simulink model "StateSpaceToScopes"  (R2023b)
settings: Solver=VariableStepAuto  StartTime=0.0  StopTime=100  RelTol=1e-3
undefined symbols (not defined in the file or in its folder): A_1, A_2, A_3, A_4, A_5, A_6, A_7, A_8, B_1, B_2, B_3, B_4, B_5, B_6, B_7, B_8, C_1, C_2, C_3, C_4, C_5, C_6, C_7, C_8, D_1, D_2, D_3, D_4, D_5, D_6, D_7, D_8, F1, F2, F3, F4, F5, F6, F7, F8, G1, G2, G3, G4, G5, G6, G7, G8, H1, H2, H3, H4, H5, H6, H7, H8, J1, J2, J3, J4 ... (+4)
settings Model: Creator=Alex  LastModifiedBy=Alex

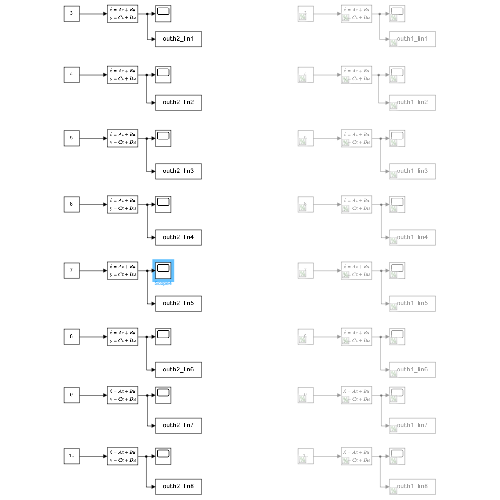
[thumbnail: Simulink's stored preview of the top-level diagram]
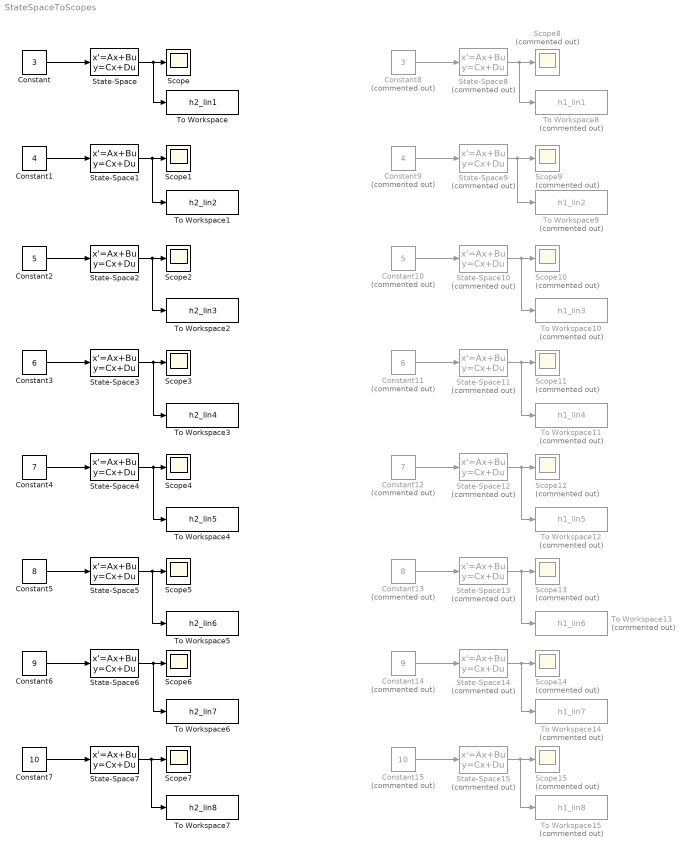
== system StateSpaceToScopes ==
  Constant : Constant  Value=3
  Constant1 : Constant  Value=4
  Constant10 : Constant  Commented=on  Value=5
  Constant11 : Constant  Commented=on  Value=6
  Constant12 : Constant  Commented=on  Value=7
  Constant13 : Constant  Commented=on  Value=8
  Constant14 : Constant  Commented=on  Value=9
  Constant15 : Constant  Commented=on  Value=10
  Constant2 : Constant  Value=5
  Constant3 : Constant  Value=6
  Constant4 : Constant  Value=7
  Constant5 : Constant  Value=8
  Constant6 : Constant  Value=9
  Constant7 : Constant  Value=10
  Constant8 : Constant  Commented=on  Value=3
  Constant9 : Constant  Commented=on  Value=4
  Scope{,1..7} (8 alike) : Scope
  Scope{8..15} (8 alike) : Scope  Commented=on
  State-Space : StateSpace  A=F1  B=G1  C=H1  D=J1  InitialCondition=0
  State-Space1 : StateSpace  A=F2  B=G2  C=H2  D=J2  InitialCondition=0
  State-Space10 : StateSpace  Commented=on  A=A_3  B=B_3  C=C_3  D=D_3  InitialCondition=0
  State-Space11 : StateSpace  Commented=on  A=A_4  B=B_4  C=C_4  D=D_4  InitialCondition=0
  State-Space12 : StateSpace  Commented=on  A=A_5  B=B_5  C=C_5  D=D_5  InitialCondition=0
  State-Space13 : StateSpace  Commented=on  A=A_6  B=B_6  C=C_6  D=D_6  InitialCondition=0
  State-Space14 : StateSpace  Commented=on  A=A_7  B=B_7  C=C_7  D=D_7  InitialCondition=0
  State-Space15 : StateSpace  Commented=on  A=A_8  B=B_8  C=C_8  D=D_8  InitialCondition=0
  State-Space2 : StateSpace  A=F3  B=G3  C=H3  D=J3  InitialCondition=0
  State-Space3 : StateSpace  A=F4  B=G4  C=H4  D=J4  InitialCondition=0
  State-Space4 : StateSpace  A=F5  B=G5  C=H5  D=J5  InitialCondition=0
  State-Space5 : StateSpace  A=F6  B=G6  C=H6  D=J6  InitialCondition=0
  State-Space6 : StateSpace  A=F7  B=G7  C=H7  D=J7  InitialCondition=0
  State-Space7 : StateSpace  A=F8  B=G8  C=H8  D=J8  InitialCondition=0
  State-Space8 : StateSpace  Commented=on  A=A_1  B=B_1  C=C_1  D=D_1  InitialCondition=0
  State-Space9 : StateSpace  Commented=on  A=A_2  B=B_2  C=C_2  D=D_2  InitialCondition=0
  To Workspace : ToWorkspace  VariableName=h2_lin1  SampleTime=-1
  To Workspace1 : ToWorkspace  VariableName=h2_lin2  SampleTime=-1
  To Workspace10 : ToWorkspace  Commented=on  VariableName=h1_lin3  SampleTime=-1
  To Workspace11 : ToWorkspace  Commented=on  VariableName=h1_lin4  SampleTime=-1
  To Workspace12 : ToWorkspace  Commented=on  VariableName=h1_lin5  SampleTime=-1
  To Workspace13 : ToWorkspace  Commented=on  VariableName=h1_lin6  SampleTime=-1
  To Workspace14 : ToWorkspace  Commented=on  VariableName=h1_lin7  SampleTime=-1
  To Workspace15 : ToWorkspace  Commented=on  VariableName=h1_lin8  SampleTime=-1
  To Workspace2 : ToWorkspace  VariableName=h2_lin3  SampleTime=-1
  To Workspace3 : ToWorkspace  VariableName=h2_lin4  SampleTime=-1
  To Workspace4 : ToWorkspace  VariableName=h2_lin5  SampleTime=-1
  To Workspace5 : ToWorkspace  VariableName=h2_lin6  SampleTime=-1
  To Workspace6 : ToWorkspace  VariableName=h2_lin7  SampleTime=-1
  To Workspace7 : ToWorkspace  VariableName=h2_lin8  SampleTime=-1
  To Workspace8 : ToWorkspace  Commented=on  VariableName=h1_lin1  SampleTime=-1
  To Workspace9 : ToWorkspace  Commented=on  VariableName=h1_lin2  SampleTime=-1
  wires:
  Constant/1 -> State-Space/1
  State-Space/1 -> To Workspace/1, Scope/1
  State-Space1/1 -> To Workspace1/1, Scope1/1
  Constant1/1 -> State-Space1/1
  State-Space2/1 -> To Workspace2/1, Scope2/1
  Constant2/1 -> State-Space2/1
  State-Space3/1 -> To Workspace3/1, Scope3/1
  Constant3/1 -> State-Space3/1
  State-Space4/1 -> To Workspace4/1, Scope4/1
  Constant4/1 -> State-Space4/1
  State-Space5/1 -> To Workspace5/1, Scope5/1
  Constant5/1 -> State-Space5/1
  State-Space6/1 -> To Workspace6/1, Scope6/1
  Constant6/1 -> State-Space6/1
  State-Space7/1 -> To Workspace7/1, Scope7/1
  Constant7/1 -> State-Space7/1
  Constant9/1 -> State-Space9/1
  Constant13/1 -> State-Space13/1
  Constant14/1 -> State-Space14/1
  State-Space14/1 -> To Workspace14/1, Scope14/1
  State-Space15/1 -> To Workspace15/1, Scope15/1
  Constant15/1 -> State-Space15/1
  State-Space10/1 -> To Workspace10/1, Scope10/1
  Constant11/1 -> State-Space11/1
  State-Space11/1 -> To Workspace11/1, Scope11/1
  State-Space8/1 -> To Workspace8/1, Scope8/1
  Constant8/1 -> State-Space8/1
  State-Space9/1 -> To Workspace9/1, Scope9/1
  State-Space13/1 -> To Workspace13/1, Scope13/1
  Constant10/1 -> State-Space10/1
  State-Space12/1 -> To Workspace12/1, Scope12/1
  Constant12/1 -> State-Space12/1
